simulink model "model_jxz"  (Simulink 7.8)
settings: Solver=FixedStepDiscrete  StartTime=0.0  StopTime=10.0  RelTol=1e-3
settings Model: Creator=jxzhang  LastModifiedBy=jxzhang
settings OptimizationCC: InlineParams=on  OptimizeModelRefInitCode=on  LifeSpan=1
settings HardwareCC: ProdIntDivRoundTo=Zero  ProdEndianess=LittleEndian  ProdHWDeviceType=Generic->Custom  TargetIntDivRoundTo=Zero  TargetEndianess=LittleEndian  TargetHWDeviceType=Generic->Custom
settings RTWCC: SystemTargetFile=tlmgenerator.tlc  GenCodeOnly=on  GenerateMakefile=off  TemplateMakefile=ert_default_tmf  PostCodeGenCommand=tlmgenerator_make_rtw_hook('post_code_gen', modelName, '', '', '', '', buildInfo)  Description=SystemC TLM Component Generator  GenerateReport=on  ProcessScript=tlmgenerator_make_rtw_hook  IncludeHyperlinkInReport=on  LaunchReport=on  TargetLang=C++  GenerateTraceInfo=on  GenerateTraceReport=on  GenerateTraceReportSl=on  GenerateTraceReportSf=on  GenerateTraceReportEml=on  GenerateCodeInfo=on
settings CodeAppCC: ForceParamTrailComments=on  IgnoreCustomStorageClasses=off  MATLABSourceComments=on
settings TLMTargetCC: TargetFcnLib=ansi_tfl_table_tmw.mat  TargetFunctionLibrary=C99 (ISO)  UtilityFuncGeneration=Auto  ERTMultiwordTypeDef=System defined  CodeExecutionProfiling=off  ERTMultiwordLength=256  MultiwordLength=2048  GenerateFullHeader=on  GenerateSampleERTMain=off  GenerateTestInterfaces=off  IsPILTarget=off  ModelReferenceCompliant=on  ParMdlRefBuildCompliant=on  CompOptLevelCompliant=off  ConcurrentExecutionCompliant=off  IncludeMdlTerminateFcn=on  GeneratePreprocessorConditionals=Use local settings  CombineOutputUpdateFcns=on  CombineSignalStateStructs=off  SuppressErrorStatus=off  ERTFirstTimeCompliant=on  IncludeFileDelimiter=Auto  ERTCustomFileBanners=on  SupportAbsoluteTime=on  LogVarNameModifier=rt_  MatFileLogging=off  MultiInstanceERTCode=on  SupportNonFinite=on  SupportComplex=on  PurelyIntegerCode=off  SupportContinuousTime=off  SupportNonInlinedSFcns=off  SupportVariableSizeSignals=off  EnableShiftOperators=on  ParenthesesLevel=Nominal  PortableWordSizes=off  ModelStepFunctionPrototypeControlCompliant=on  CPPClassGenCompliant=on  AutosarCompliant=off  GenerateErtSFunction=off  CreateSILPILBlock=None  CodeExecutionProfileVariable=executionProfile  CodeProfilingSaveOptions=SummaryOnly  GenerateASAP2=off  ExtMode=off  ExtModeTransport=0  ExtModeStaticAlloc=off  ExtModeStaticAllocSize=1000000  ExtModeTesting=off  ExtModeMexFile=noextcomm  ExtModeIntrfLevel=Level1  InlinedParameterPlacement=Hierarchical  TargetOS=BareBoardExample  MultiInstanceErrorCode=Error  RateGroupingCode=on  RootIOFormat=Structure reference  RTWCAPISignals=off  RTWCAPIParams=off  RTWCAPIStates=off  RTWCAPIRootIO=off  ERTSrcFileBannerTemplate=ert_code_template.cgt  ERTHdrFileBannerTemplate=ert_code_template.cgt  ERTDataSrcFileTemplate=ert_code_template.cgt  ERTDataHdrFileTemplate=ert_code_template.cgt  ERTCustomFileTemplate=example_file_process.tlc  CoverageDialogOpen=off  EnableDataOwnership=off  SignalDisplayLevel=10  ParamTuneLevel=10  GlobalDataDefinition=Auto  DataDefinitionFile=global.c  GlobalDataReference=Auto  ERTFilePackagingFormat=Modular  DataReferenceFile=global.h  GRTInterface=off  PreserveExpressionOrder=off  PreserveIfCondition=off  ConvertIfToSwitch=off  PreserveExternInFcnDecls=on  SuppressUnreachableDefaultCases=off  EnableUserReplacementTypes=off  MemSecPackage=--- None ---  MemSecDataConstants=Default  MemSecDataIO=Default  MemSecDataInternal=Default  MemSecDataParameters=Default  MemSecFuncInitTerm=Default  MemSecFuncExecute=Default  MemSecFuncSharedUtil=Default  CodeProfilingInstrumentation=off  tlmgComponentAddressing=No memory map  tlmgAutoAddressSpecType=Single input and output address offsets  tlmgCommandStatusRegOnOff=off  tlmgTestAndSetRegOnOff=off  tlmgProcessingType=SystemC Thread  tlmgIrqPortOnOff=on  tlmgPayloadBufferingOnOff=off  tlmgPayloadInBufferDepth=1  tlmgPayloadOutBufferDepth=1  tlmgTempDecouplOnOff=off  tlmgMaxQuantumTime=1000  tlmgAlgorithmProcessingTime=100  tlmgFirstWriteTime=10  tlmgSubsequentWritesInBurstTime=10  tlmgFirstReadTime=10  tlmgSubsequentReadsInBurstTime=10  tlmgGenerateTestbenchOnOff=on  tlmgVerboseTbMessagesOnOff=off  tlmgRuntimeTimingMode=With timing  tlmgInputBufferTriggerMode=Automatic  tlmgOutputBufferTriggerMode=Automatic  tlmgKeepInputBufferFullOnOff=on  tlmgKeepOutputBufferFullOnOff=on  tlmgSystemCIncludePath=$(SYSTEMC_INC_PATH)  tlmgSystemCLibPath=$(SYSTEMC_LIB_PATH)  tlmgSystemCLibName=$(SYSTEMC_LIB_NAME)  tlmgTLMIncludePath=$(TLM_INC_PATH)  tlmgTbExeDir=model_jxz_VP/model_jxz_tlm_tb  tlmgTbNumVectors=0

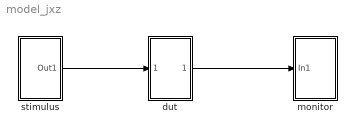
== system model_jxz ==
  dut : Subsystem
  monitor : Subsystem
  stimulus : Subsystem
  wires:
  dut/1(Out1) -> monitor/1(In1)
  stimulus/1(Out1) -> dut/1(In1)

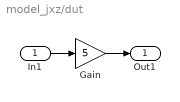
== system model_jxz/dut ==
  In1 : Inport
  Gain : Gain  Gain=5
  Out1 : Outport
  wires:
  In1/1 -> Gain/1
  Gain/1 -> Out1/1

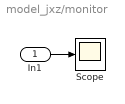
== system model_jxz/monitor ==
  In1 : Inport
  Scope : Scope
  wires:
  In1/1 -> Scope/1

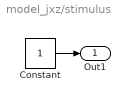
== system model_jxz/stimulus ==
  Constant : Constant
  Out1 : Outport
  wires:
  Constant/1 -> Out1/1
